simulink model "feedback_relative"  (R2020a)
settings: Solver=ode4  StartTime=0.0  StopTime=10  FixedStep=0.002  RelTol=1e-3
values from neighbouring files (symbols this model uses):
  A = 1    [bode_hiratsuka_damper.m]    (also in exp_dampa.m = 0.007; mf_dampa_1DOF.m = 0.003; mf_feedback_relative.m = 0.003; mf_nonlinear_relative.m = 0.01)
  Aor = 0.1*10^-6    (= 1e-07)    [bode_hiratsuka_damper.m]    (also in exp_dampa.m; mf_dampa_1DOF.m; mf_feedback_relative.m; mf_nonlinear_relative.m)
  Ap = (32.50*0.001)^2*pi/4    (= 0.000829576810089)    [bode_hiratsuka_damper.m]    (also in exp_dampa.m; mf_dampa_1DOF.m; mf_feedback_relative.m; mf_nonlinear_relative.m)
  c1 = 7    [mf_feedback_relative.m]    (also in mf_nonlinear_relative.m; mf_with_P.m; mf_with_Pm.m; mf_with_double.m)
  Cor = 0.8    [bode_hiratsuka_damper.m]    (also in exp_dampa.m; mf_dampa_1DOF.m; mf_feedback_relative.m; mf_nonlinear_relative.m)
  Hz = wv(k)    [bode_hiratsuka_damper.m]    (also in exp_dampa.m = 18.8495559215; mf_dampa_1DOF.m = 6.28318530718; mf_feedback_relative.m = 6.28318530718; mf_nonlinear_relative.m = 6.28318530718)
  k1 = 2200    [mf_dampa_1DOF.m]    (also in mf_feedback_relative.m; mf_nonlinear_relative.m; mf_with_P.m; mf_with_Pm.m)
  k2 = 405    [mf_dampa_1DOF.m]    (also in mf_feedback_relative.m; mf_nonlinear_relative.m; mf_with_P.m; mf_with_Pm.m)
  kappa = 1.4    [bode_hiratsuka_damper.m]    (also in exp_dampa.m; mf_dampa_1DOF.m; mf_feedback_relative.m; mf_nonlinear_relative.m)
  m1 = 1.5    [mf_dampa_1DOF.m]    (also in mf_feedback_relative.m; mf_nonlinear_relative.m; mf_with_P.m; mf_with_Pm.m)
  m2 = 6.4    [mf_feedback_relative.m]    (also in mf_nonlinear_relative.m; mf_with_P.m; mf_with_Pm.m; mf_with_double.m)
  P0 = 101325    [bode_hiratsuka_damper.m]    (also in exp_dampa.m; mf_dampa_1DOF.m; mf_feedback_relative.m; mf_nonlinear_relative.m)
  row0 = 1.1841    [bode_hiratsuka_damper.m]    (also in exp_dampa.m; mf_dampa_1DOF.m; mf_feedback_relative.m; mf_nonlinear_relative.m)
  x0 = 0.05    [bode_hiratsuka_damper.m]    (also in exp_dampa.m = 0.042; mf_dampa_1DOF.m = 0.042; mf_feedback_relative.m = 0.042; mf_nonlinear_relative.m = 0.042)
settings Model: Creator=Peanatsu  LastModifiedBy=Peanatsu

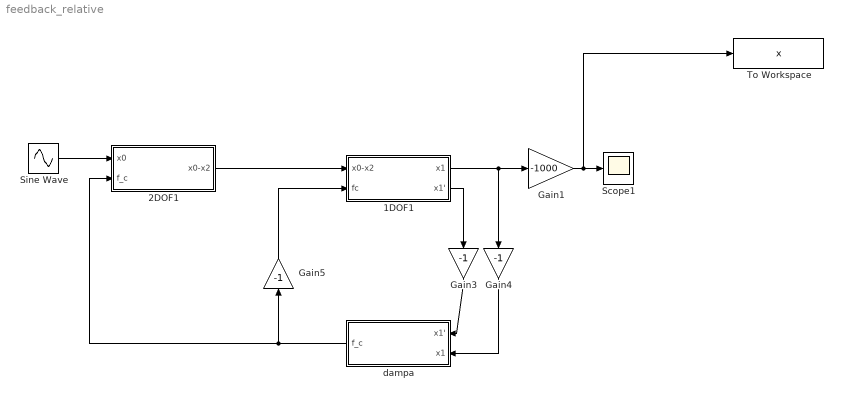
== system feedback_relative ==
  1DOF1 : Subsystem
  2DOF1 : Subsystem
  Gain1 : Gain  Gain=-1000
  Gain3 : Gain  Gain=-1
  Gain4 : Gain  Gain=-1
  Gain5 : Gain  Gain=-1
  Scope1 : Scope
  Sine Wave : Sin  Amplitude=A  Frequency=Hz  SampleTime=0
  To Workspace : ToWorkspace  VariableName=x  SaveFormat=Timeseries  SampleTime=-1
  dampa : Subsystem
  wires:
  2DOF1/1(x0-x2) -> 1DOF1/1(x0-x2)
  Sine Wave/1 -> 2DOF1/1(x0)
  1DOF1/1(x1) -> Gain4/1, Gain1/1
  Gain1/1 -> To Workspace/1, Scope1/1
  1DOF1/2(x1') -> Gain3/1
  Gain3/1 -> dampa/1(x1')
  Gain4/1 -> dampa/2(x1)
  dampa/1(f_c) -> 2DOF1/2(f_c), Gain5/1
  Gain5/1 -> 1DOF1/2(fc)

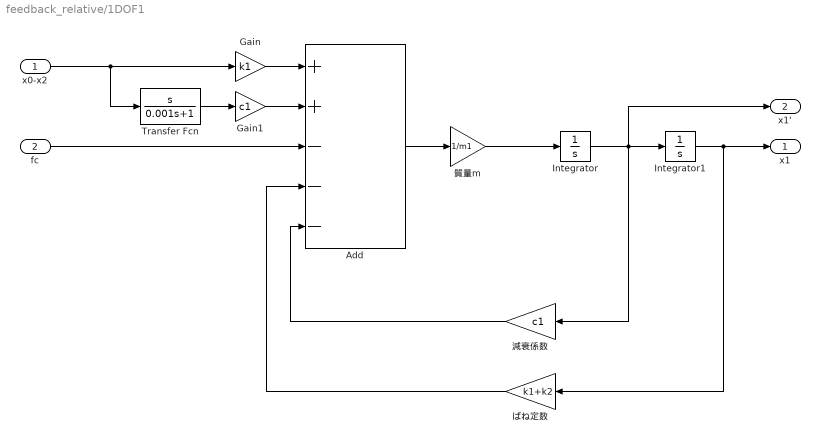
== system feedback_relative/1DOF1 ==
  x0-x2 : Inport
  fc : Inport  Port=2
  Add : Sum  Inputs=++---
  Gain : Gain  Gain=k1
  Gain1 : Gain  Gain=c1
  Integrator : Integrator
  Integrator1 : Integrator
  Transfer Fcn : TransferFcn  Numerator=[1 0]  Denominator=[0.001 1]
  "ばね定数 " : Gain  Gain=k1+k2
  減衰係数 : Gain  Gain=c1
  質量m : Gain  Gain=1/m1
  x1 : Outport
  x1' : Outport  Port=2
  wires:
  Integrator/1 -> 減衰係数/1, x1'/1, Integrator1/1
  Add/1 -> 質量m/1
  x0-x2/1 -> Transfer Fcn/1, Gain/1
  質量m/1 -> Integrator/1
  Integrator1/1 -> x1/1, "ばね定数 "/1
  Gain/1 -> Add/1
  Gain1/1 -> Add/2
  Transfer Fcn/1 -> Gain1/1
  減衰係数/1 -> Add/5
  "ばね定数 "/1 -> Add/4
  fc/1 -> Add/3

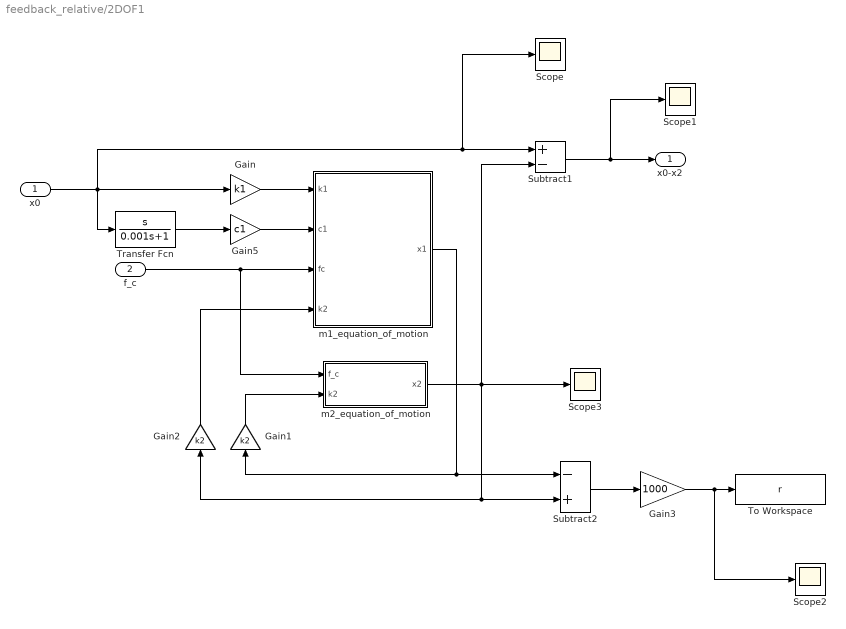
== system feedback_relative/2DOF1 ==
  x0 : Inport
  f_c : Inport  Port=2
  Gain : Gain  Gain=k1
  Gain1 : Gain  Gain=k2
  Gain2 : Gain  Gain=k2
  Gain3 : Gain  Gain=1000
  Gain5 : Gain  Gain=c1
  Scope{,1..3} (4 alike) : Scope
  Subtract1 : Sum  Inputs=+-
  Subtract2 : Sum  Inputs=-+
  To Workspace : ToWorkspace  VariableName=r  SaveFormat=Timeseries  SampleTime=-1
  Transfer Fcn : TransferFcn  Numerator=[1 0]  Denominator=[0.001 1]
  m1_equation_of_motion : Subsystem
  m2_equation_of_motion : Subsystem
  x0-x2 : Outport
  wires:
  x0/1 -> Transfer Fcn/1, Scope/1, Subtract1/1, Gain/1
  Gain/1 -> m1_equation_of_motion/1(k1)
  m1_equation_of_motion/1(x1) -> Subtract2/1, Gain1/1
  Subtract1/1 -> Scope1/1, x0-x2/1
  Gain1/1 -> m2_equation_of_motion/2("k2 ")
  Subtract2/1 -> Gain3/1
  Gain3/1 -> Scope2/1, To Workspace/1
  m2_equation_of_motion/1(x2) -> Scope3/1, Gain2/1, Subtract2/2, Subtract1/2
  Gain2/1 -> m1_equation_of_motion/4(k2)
  f_c/1 -> m2_equation_of_motion/1(f_c), m1_equation_of_motion/3(fc)
  Gain5/1 -> m1_equation_of_motion/2(c1)
  Transfer Fcn/1 -> Gain5/1

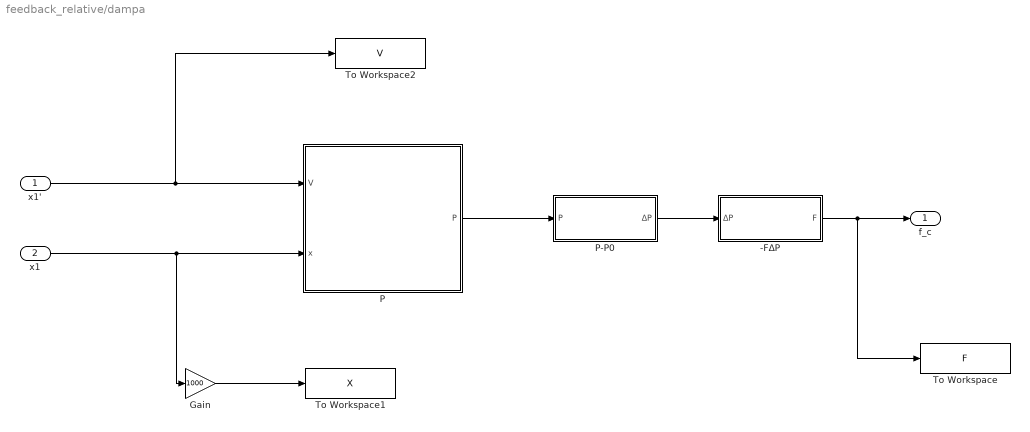
== system feedback_relative/dampa ==
  x1' : Inport
  x1 : Inport  Port=2
  -FΔP : Subsystem
  Gain : Gain  Gain=1000
  P : Subsystem
  P-P0 : Subsystem
  To Workspace : ToWorkspace  VariableName=F  SaveFormat=Timeseries  SampleTime=-1
  To Workspace1 : ToWorkspace  VariableName=X  SaveFormat=Timeseries  SampleTime=-1
  To Workspace2 : ToWorkspace  VariableName=V  SaveFormat=Timeseries  SampleTime=-1
  f_c : Outport
  wires:
  x1'/1 -> To Workspace2/1, P/1(V)
  P/1(P) -> P-P0/1(P)
  P-P0/1(ΔP) -> -FΔP/1(ΔP)
  x1/1 -> Gain/1, P/2(x)
  -FΔP/1(F) -> To Workspace/1, f_c/1
  Gain/1 -> To Workspace1/1

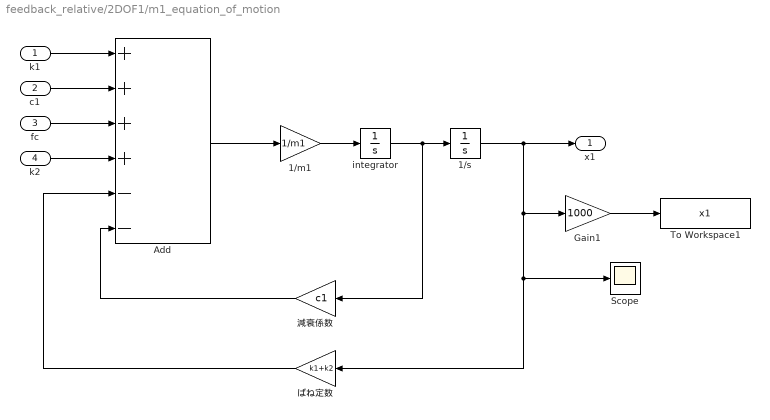
== system feedback_relative/2DOF1/m1_equation_of_motion ==
  k1 : Inport
  c1 : Inport  Port=2
  fc : Inport  Port=3
  k2 : Inport  Port=4
  1/m1 : Gain  Gain=1/m1
  1/s : Integrator
  Add : Sum  Inputs=++++--
  Gain1 : Gain  Gain=1000
  Scope : Scope
  To Workspace1 : ToWorkspace  VariableName=x1  SaveFormat=Timeseries  SampleTime=-1
  integrator : Integrator
  ばね定数 : Gain  Gain=k1+k2
  減衰係数 : Gain  Gain=c1
  x1 : Outport
  wires:
  k1/1 -> Add/1
  Add/1 -> 1/m1/1
  integrator/1 -> 減衰係数/1, 1/s/1
  1/s/1 -> x1/1, Gain1/1, Scope/1, ばね定数/1
  1/m1/1 -> integrator/1
  Gain1/1 -> To Workspace1/1
  ばね定数/1 -> Add/5
  c1/1 -> Add/2
  fc/1 -> Add/3
  k2/1 -> Add/4
  減衰係数/1 -> Add/6

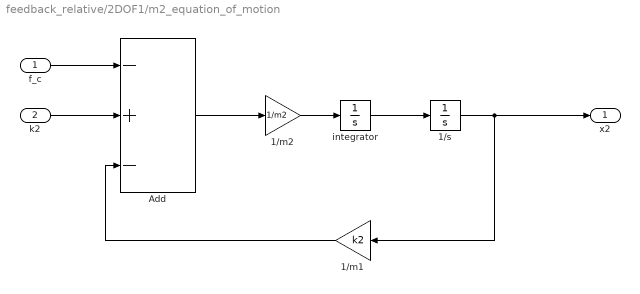
== system feedback_relative/2DOF1/m2_equation_of_motion ==
  f_c : Inport
  "k2 " : Inport  Port=2
  1/m1 : Gain  Gain=k2
  1/m2 : Gain  Gain=1/m2
  1/s : Integrator
  Add : Sum  Inputs=-+-
  integrator : Integrator
  x2 : Outport
  wires:
  f_c/1 -> Add/1
  "k2 "/1 -> Add/2
  Add/1 -> 1/m2/1
  integrator/1 -> 1/s/1
  1/s/1 -> 1/m1/1, x2/1
  1/m1/1 -> Add/3
  1/m2/1 -> integrator/1

== system feedback_relative/dampa/-FΔP ==
  ΔP : Inport
  Constant : Constant  Value=Ap
  Product : Product
  F : Outport
  wires:
  Constant/1 -> Product/2
  ΔP/1 -> Product/1
  Product/1 -> F/1

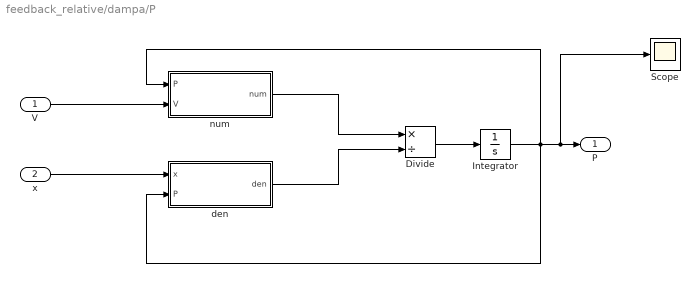
== system feedback_relative/dampa/P ==
  V : Inport
  x : Inport  Port=2
  Divide : Product  Inputs=*/
  Integrator : Integrator  InitialCondition=P0
  Scope : Scope
  den : Subsystem
  num : Subsystem
  P : Outport
  wires:
  Integrator/1 -> Scope/1, P/1, num/1(P), den/2(P)
  V/1 -> num/2(V)
  Divide/1 -> Integrator/1
  x/1 -> den/1(x)
  den/1(den) -> Divide/2
  num/1(num) -> Divide/1

== system feedback_relative/dampa/P-P0 ==
  P : Inport
  Add : Sum  Inputs=+-
  Constant : Constant  Value=P0
  ΔP : Outport
  wires:
  P/1 -> Add/1
  Constant/1 -> Add/2
  Add/1 -> ΔP/1

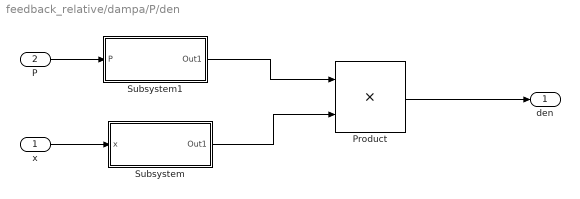
== system feedback_relative/dampa/P/den ==
  x : Inport
  P : Inport  Port=2
  Product : Product
  Subsystem : Subsystem
  Subsystem1 : Subsystem
  den : Outport
  wires:
  x/1 -> Subsystem/1(x)
  P/1 -> Subsystem1/1(P)
  Subsystem1/1(Out1) -> Product/1
  Subsystem/1(Out1) -> Product/2
  Product/1 -> den/1

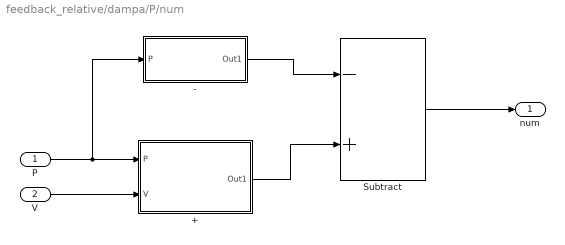
== system feedback_relative/dampa/P/num ==
  P : Inport
  V : Inport  Port=2
  + : Subsystem
  - : Subsystem
  Subtract : Sum  Inputs=-+
  num : Outport
  wires:
  V/1 -> +/2(V)
  P/1 -> -/1(P), +/1(P)
  +/1(Out1) -> Subtract/2
  -/1(Out1) -> Subtract/1
  Subtract/1 -> num/1

== system feedback_relative/dampa/P/den/Subsystem ==
  x : Inport
  Add : Sum  Inputs=+-
  Constant1 : Constant
  Gain : Gain  Gain=1/x0
  Out1 : Outport
  wires:
  Gain/1 -> Add/2
  Constant1/1 -> Add/1
  Add/1 -> Out1/1
  x/1 -> Gain/1

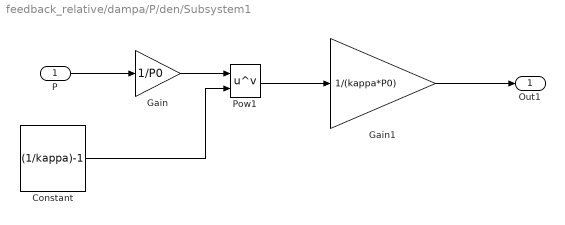
== system feedback_relative/dampa/P/den/Subsystem1 ==
  P : Inport
  Constant : Constant  Value=(1/kappa)-1
  Gain : Gain  Gain=1/P0
  Gain1 : Gain  Gain=1/(kappa*P0)
  Pow1 : Math  Operator=pow  SignedPower=on  OutputSignalType=real  SaturateOnIntegerOverflow=on
  Out1 : Outport
  wires:
  P/1 -> Gain/1
  Gain/1 -> Pow1/1
  Constant/1 -> Pow1/2
  Gain1/1 -> Out1/1
  Pow1/1 -> Gain1/1

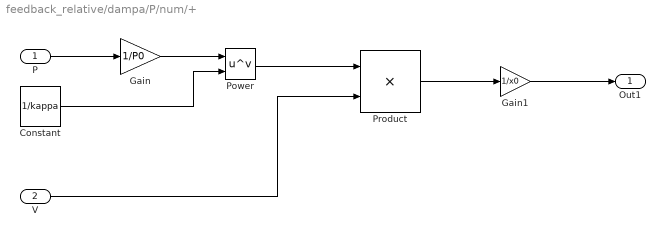
== system feedback_relative/dampa/P/num/+ ==
  P : Inport
  V : Inport  Port=2
  Constant : Constant  Value=1/kappa
  Gain : Gain  Gain=1/P0
  Gain1 : Gain  Gain=1/x0
  Power : Math  Operator=pow  SignedPower=on  OutputSignalType=real  SaturateOnIntegerOverflow=on
  Product : Product
  Out1 : Outport
  wires:
  Gain/1 -> Power/1
  Constant/1 -> Power/2
  Power/1 -> Product/1
  V/1 -> Product/2
  Gain1/1 -> Out1/1
  Product/1 -> Gain1/1
  P/1 -> Gain/1

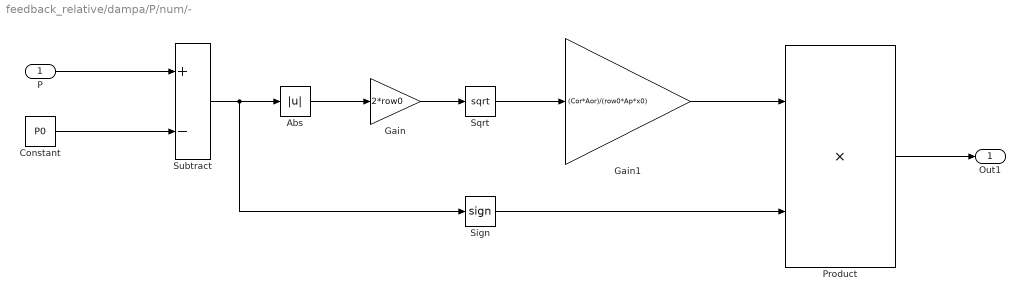
== system feedback_relative/dampa/P/num/- ==
  P : Inport
  Abs : Abs
  Constant : Constant  Value=P0
  Gain : Gain  Gain=2*row0
  Gain1 : Gain  Gain=(Cor*Aor)/(row0*Ap*x0)
  Product : Product
  Sign : Signum
  Sqrt : Sqrt  SaturateOnIntegerOverflow=on
  Subtract : Sum  Inputs=+-
  Out1 : Outport
  wires:
  Abs/1 -> Gain/1
  Gain/1 -> Sqrt/1
  Sqrt/1 -> Gain1/1
  Sign/1 -> Product/2
  Gain1/1 -> Product/1
  Product/1 -> Out1/1
  Subtract/1 -> Sign/1, Abs/1
  P/1 -> Subtract/1
  Constant/1 -> Subtract/2
